simulink model "Proiect_EP"  (R2024b)
settings: Solver=VariableStepAuto  StartTime=0.0  StopTime=10.0  RelTol=1e-3
values from neighbouring files (symbols this model uses):
  C = 2.56e-3    (= 0.00256)    [P4.m]    (also in Proiect3_1.m = 0.00078125; ProiectEP_3.m = 0.00078125; ProiectEP_Init.m = 0.00078125; Proiect_2.m = 0.00078125)
  Cr = 0.00001    (= 1e-05)    [ProiectEP_Init.m]
  L = 2.944e-3    (= 0.002944)    [P4.m]    (also in Proiect3_1.m = 0.001405155; ProiectEP_3.m = 0.001405155; ProiectEP_Init.m = 0.001405155; Proiect_2.m = 0.001405155)
  Lr = 0.002    [ProiectEP_Init.m]
  R = 0.1    [P4.m]    (also in Proiect3_1.m = 0.4; ProiectEP_3.m = 0.4; ProiectEP_Init.m = 0.4; Proiect_2.m = 0.4)
  Uin = 48    [P4.m]    (also in Proiect3_1.m; ProiectEP_3.m; ProiectEP_Init.m; Proiect_2.m)
settings Model: Creator=Razvan  LastModifiedBy=Razvan

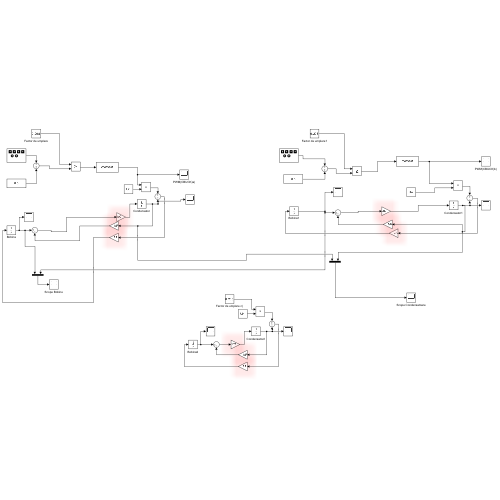
[thumbnail: Simulink's stored preview of the top-level diagram]
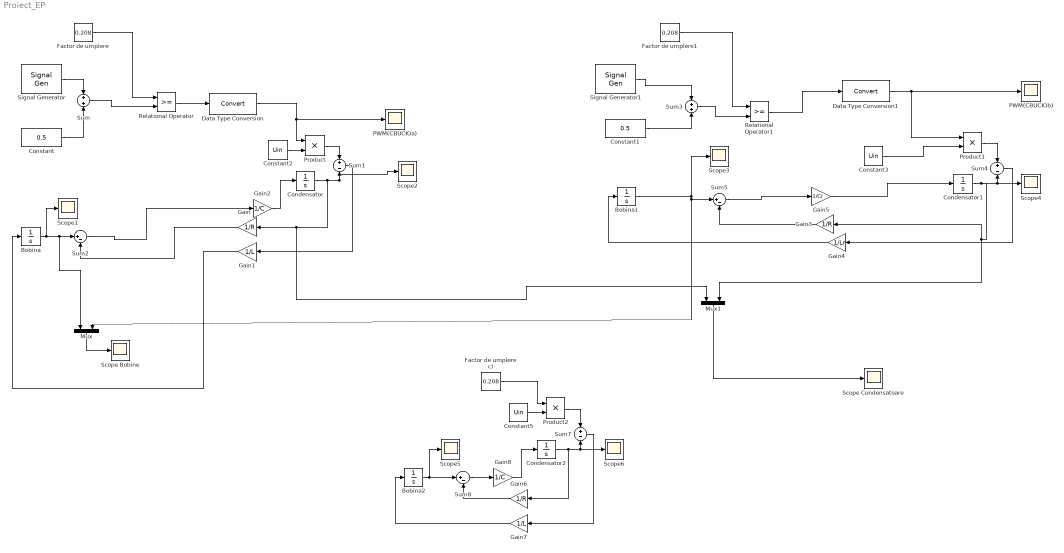
== system Proiect_EP ==
  Bobina : Integrator
  Bobina1 : Integrator
  Bobina2 : Integrator
  Condensator : Integrator
  Condensator1 : Integrator
  Condensator2 : Integrator
  Constant : Constant  Value=0.5
  Constant1 : Constant  Value=0.5
  Constant2 : Constant  Value=Uin
  Constant3 : Constant  Value=Uin
  Constant5 : Constant  Value=Uin
  Data Type Conversion : DataTypeConversion  SaturateOnIntegerOverflow=off  RndMeth=Floor
  Data Type Conversion1 : DataTypeConversion  SaturateOnIntegerOverflow=off  RndMeth=Floor
  Factor de umplere : Constant  Value=0.208
  Factor de umplere c) : Constant  Value=0.208
  Factor de umplere1 : Constant  Value=0.208
  Gain : Gain  Gain=1/R
  Gain1 : Gain  Gain=1/L
  Gain2 : Gain  Gain=1/C
  Gain3 : Gain  Gain=1/R
  Gain4 : Gain  Gain=1/Lr
  Gain5 : Gain  Gain=1/Cr
  Gain6 : Gain  Gain=1/R
  Gain7 : Gain  Gain=1/L
  Gain8 : Gain  Gain=1/C
  Mux : Mux  Inputs=2
  Mux1 : Mux  Inputs=2
  PWM(CBUCK)a) : Scope
  PWM(CBUCK)b) : Scope
  Product : Product  Inputs=**
  Product1 : Product  Inputs=**
  Product2 : Product  Inputs=**
  Relational Operator : RelationalOperator  OutDataTypeStr=boolean  RndMeth=Simplest  InputSameDT=off
  Relational Operator1 : RelationalOperator  OutDataTypeStr=boolean  RndMeth=Simplest  InputSameDT=off
  Scope Bobine : Scope
  Scope Condensatoare : Scope
  Scope{1..6} (6 alike) : Scope
  Signal Generator : SignalGenerator  WaveForm=sawtooth  Amplitude=0.5  Frequency=1500
  Signal Generator1 : SignalGenerator  WaveForm=sawtooth  Amplitude=0.5  Frequency=1500
  Sum : Sum
  Sum1 : Sum  Inputs=+-
  Sum2 : Sum  Inputs=|+-
  Sum3 : Sum
  Sum4 : Sum  Inputs=+-
  Sum5 : Sum  Inputs=|+-
  Sum7 : Sum  Inputs=+-
  Sum8 : Sum  Inputs=|+-
  wires:
  Gain5/1 -> Condensator1/1
  Product/1 -> Sum1/1
  Signal Generator1/1 -> Sum3/1
  Constant3/1 -> Product1/2
  Sum7/1 -> Gain7/1
  Data Type Conversion/1 -> PWM(CBUCK)a)/1, Product/1
  Mux/1 -> Scope Bobine/1
  Sum2/1 -> Gain2/1
  Factor de umplere1/1 -> Relational Operator1/1
  Sum/1 -> Relational Operator/2
  Constant2/1 -> Product/2
  Gain2/1 -> Condensator/1
  Product2/1 -> Sum7/1
  Constant1/1 -> Sum3/2
  Factor de umplere/1 -> Relational Operator/1
  Sum4/1 -> Gain4/1
  Gain4/1 -> Bobina1/1
  Condensator/1 -> Sum1/2, Scope2/1, Mux1/1, Gain/1
  Sum5/1 -> Gain5/1
  Data Type Conversion1/1 -> Product1/1, PWM(CBUCK)b)/1
  Constant/1 -> Sum/2
  Sum8/1 -> Gain8/1
  Signal Generator/1 -> Sum/1
  Sum1/1 -> Gain1/1
  Gain1/1 -> Bobina/1
  Bobina1/1 -> Mux/2, Sum5/1, Scope3/1
  Relational Operator1/1 -> Data Type Conversion1/1
  Condensator1/1 -> Sum4/2, Scope4/1, Mux1/2, Gain3/1
  Relational Operator/1 -> Data Type Conversion/1
  Bobina2/1 -> Sum8/1, Scope5/1
  Mux1/1 -> Scope Condensatoare/1
  Product1/1 -> Sum4/1
  Gain6/1 -> Sum8/2
  Condensator2/1 -> Sum7/2, Scope6/1, Gain6/1
  Gain/1 -> Sum2/2
  Factor de umplere c)/1 -> Product2/1
  Constant5/1 -> Product2/2
  Gain7/1 -> Bobina2/1
  Gain3/1 -> Sum5/2
  Sum3/1 -> Relational Operator1/2
  Bobina/1 -> Sum2/1, Mux/1, Scope1/1
  Gain8/1 -> Condensator2/1
